simulink model "CalculatorChart_GraphicalFunc"  (R2017b)
settings: Solver=FixedStepDiscrete  StartTime=0.0  StopTime=10.0  RelTol=1e-3
settings Model: Creator=engdo  LastModifiedBy=engdo
settings OptimizationCC: DefaultParameterBehavior=Inlined  PassReuseOutputArgsAs=Individual arguments
settings DebuggingCC: ParameterTunabilityLossMsg=error
settings SFSimCC: MATLABDynamicMemAlloc=off
settings RTWCC: SystemTargetFile=ert.tlc  GenCodeOnly=on  TemplateMakefile=ert_default_tmf  GenerateReport=on  IncludeHyperlinkInReport=on  LaunchReport=on  GenerateTraceInfo=on  GenerateTraceReport=on  GenerateTraceReportSl=on  GenerateTraceReportSf=on  GenerateTraceReportEml=on  GenerateWebview=on
settings CodeAppCC: ForceParamTrailComments=on  IgnoreCustomStorageClasses=off  OperatorAnnotations=on  SimulinkDataObjDesc=on  SFDataObjDesc=on  InsertBlockDesc=on
settings ERTTargetCC: TargetLangStandard=C99 (ISO)  GenerateSampleERTMain=on  InlinedParameterPlacement=NonHierarchical  ERTCustomFileTemplate=example_file_process.tlc  EnableUserReplacementTypes=on

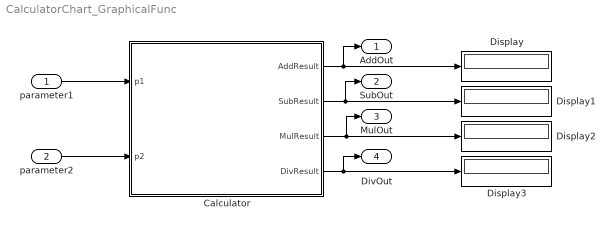
== system CalculatorChart_GraphicalFunc ==
  parameter1 : Inport
  parameter2 : Inport  Port=2
  Calculator : Stateflow chart  TreatAsAtomicUnit=on
  Display{,1..3} (4 alike) : Display
  AddOut : Outport
  SubOut : Outport  Port=2
  MulOut : Outport  Port=3
  DivOut : Outport  Port=4
  wires:
  Calculator/1(AddResult) -> AddOut/1, Display/1
  parameter1/1 -> Calculator/1(p1)
  parameter2/1 -> Calculator/2(p2)
  Calculator/2(SubResult) -> SubOut/1, Display1/1
  Calculator/3(MulResult) -> MulOut/1, Display2/1
  Calculator/4(DivResult) -> DivOut/1, Display3/1

== stateflow chart CalculatorChart_GraphicalFunc/Calculator ==
  state Result=Add(n1,n2) [function]
    (default) -> (junction 52) : {Result = n1+n2;}
  state Result=Sub(n1,n2) [function]
    (default) -> (junction 67) : {Result = n1-n2;}
  state Result=Mul(n1,n2) [function]
    (default) -> (junction 73) : {Result = n1*n2;}
  state Result=Div(n1,n2) [function]
    (default) -> (junction 79) : {Result = n1/n2;}
  (default) -> (junction 46)
  (junction 46) -> (junction 13)
  (junction 13) -> (junction 14) : {
      | AddResult =Add(p1,p2);
      | SubResult=Sub(p1,p2);
      | MulResult=Mul(p1,p2);
      | DivResult=Div(p1,p2);
      | }
  data: n1 function_input double; n2 function_input double; Result function_output double; n1 function_input double; n2 function_input double; Result function_output double; n1 function_input double; n2 function_input double; Result function_output double; n1 function_input double; n2 function_input double; Result function_output double; p1 input; p2 input; AddResult output; SubResult output; MulResult output; DivResult output
